simulink library "microgridLibrary"  (R2018b)
settings: Solver=VariableStepAuto  StartTime=0.0  StopTime=10.0  RelTol=1e-3
undefined symbols (not defined in the file): BR, D1, Delta, DiscIntNeverNeededParam, Fn, gcbh, Ion, kv, Lithium, Ls, Rs, sps_rtmsupport, StationData, Ts, Ts_Control, Vn
libraries: powerlib x80, simulink x29, powerlib_meascontrol x28, sps_avr x5, spsDieselMotorModel x3, electricdrivelib x2, re_lib x1
(part 1 of 6)
settings Model: Creator=jlesage  LastModifiedBy=jlesage
settings DebuggingCC: LibraryContextMissingDiagnostic=none
settings SFSimCC: SimUseLocalCustomCode=off
settings RTWCC: RTWUseLocalCustomCode=off

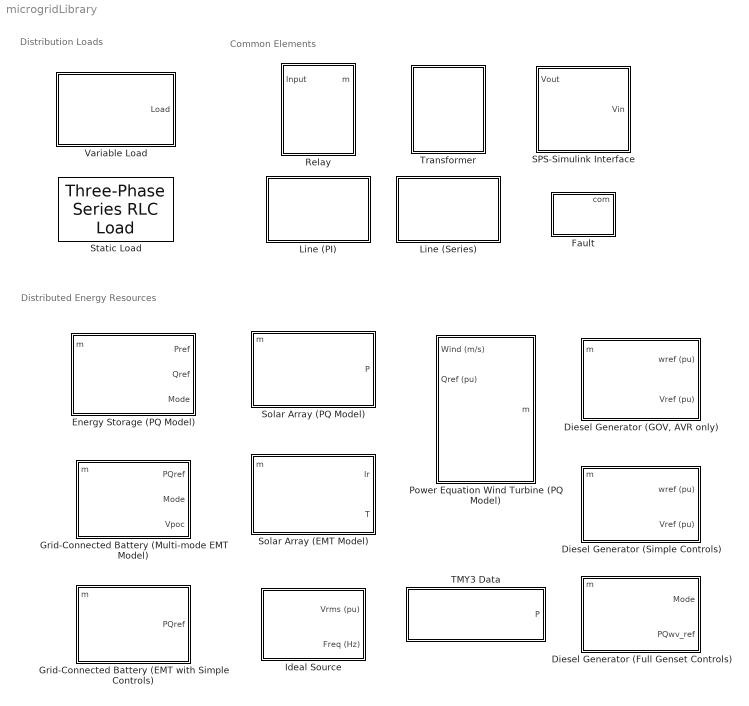
== system microgridLibrary ==
  note: Distribution Loads
  note: Common Elements
  note: Distributed Energy Resources
  Diesel Generator (Full Genset Controls) : Subsystem  VariantControlMode=Label  Variant=on  VariantControl=Variant1  LabelModeActiveChoice=Continuous  mask(Diesel Generator (Full Genset Model)){Pn=1e7, Vn=5000, Fn=60, genType=PQ, PQ0=[0.8 0], Ts=0, copyToDis=on}
      mask prompts: Pn "Generator Rated Power [W]"; Vn "Rated Voltage [V]"; Fn "Rated Frequency [Hz]"; genType "Load Flow Type"; PQ0 "Initial Power, [P0 Q0] [pu]"; Ts "Sample Time [s]"; copyToDis "Copy Load Flow to Discrete"
      mask help:
      | The Diesel Generator block contains a synchronous generator, diesel governor and excitation system to represent the dynamics of a Genset. Additional Genset controls are available for different control tasks, such as PQ control, PV control and VF control.
      |
      | The inputs to the Genset block are Mode (0 - VF control, 1 - PQ control, 2 - PV control)  and the command vector (Pref, Qref, wref, Vref) . The output measurements are contained in a Simulink bus, which can be selected by using the Bus Selector block.
      |
      | Note: The initial generator power must be specified for use for Load Flow analysis.
      mask init:
      | pf = 0.95;
      | 
      | % Extract Initial Active/Reactive Power
      | P0 = PQ0(1);
      | Q0 = PQ0(2);
      | 
      | simulationStatus =  get_param(bdroot,'SimulationStatus');
      | 
      | % The active variant can only be modified at edit-time or very early during
      | % the simulink compile stage. 
      | if any(strcmp(simulationStatus, {'stopped'}))
      |     vssBlk = gcb;
      |     oldVariant = get_param(gcb,'OverrideUsingVariant');
      | 
      |     if Ts == 0
      |         set_param(vssBlk, 'OverrideUsingVariant', 'Continuous');
      |     else
      |         set_param(vssBlk, 'OverrideUsingVariant', 'Discrete');
      |     end
      | end
      | 
      | % Select Load Flow Type
      | genBlock = [gcb '/Continuous/Synchronous Machine'];
      | currentVals = get_param(genBlock,'MaskValues');
      | currentVals{31} = genType;
      | set_param(genBlock,'MaskValues',currentVals);
      | 
      | % Disable Option if Swing Generator Selected
      | currentEnables = get_param(gcb,'MaskEnables');
      | if strcmp(genType,'swing') && Ts == 0
      |     currentEnables{4} = 'on';
      |     currentEnables{5} = 'off';
      | elseif Ts == 0
      |     currentEnables{4} = 'on';
      |     currentEnables{5} = 'on';
      | else
      |     currentEnables{4} = 'off';
      |     currentEnables{5} = 'off';
      | end
      | set_param(gcb,'MaskEnables',currentEnables);
      | 
      | % Copy Load Flow Results to Discrete
      | if copyToDis
      | contGenBlock = [gcb '/Continuous/Synchronous Machine'];
      | contGovBlock = [gcb '/Continuous/Diesel Engine Governor'];
      | contAvrBlock = [gcb '/Continuous/Excitation System'];
      | 
      | disGenBlock = [gcb '/Discrete/Synchronous Machine'];
      | disGovBlock = [gcb '/Discrete/Diesel Engine Governor'];
      | disAvrBlock = [gcb '/Discrete/Excitation System'];
      | 
      | contGenParam = get_param(contGenBlock,'MaskValues');
      | contGovParam = get_param(contGovBlock,'MaskValues');
      | contAvrParam = get_param(contAvrBlock,'MaskValues');
      | 
      | disGenParam = get_param(disGenBlock,'MaskValues');
      | disGovParam = get_param(disGovBlock,'MaskValues');
      | disAvrParam = get_param(disAvrBlock,'MaskValues');
      | 
      | % Overwrite Initial Conditions
      | disGenParam{23} = contGenParam{23};
      | disGovParam{6} = contGovParam{6};
      | disAvrParam{12} = contAvrParam{12};
      | 
      | set_param(disGenBlock,'MaskValues',disGenParam);
      | set_param(disGovBlock,'MaskValues',disGovParam);
      | set_param(disAvrBlock,'MaskValues',disAvrParam);
      | end
      mask TypeOptions genType: swing | PQ
      mask Display:
      | color('black')
      | port_label('input',1,'Mode')
      | port_label('input',2,'PQwvRef')
      | port_label('output',1,'m')
      | port_label('Rconn',1,'A')
      | port_label('Rconn',2,'B')
      | port_label('Rconn',3,'C')
  "Diesel Generator (GOV, AVR only)" : Subsystem  mask(Diesel Generator (Simple)){Pn=1e6, Vn=5000, Fn=60, genType=PQ, PQ0=[0.05 0]}
      mask prompts: Pn "Generator Rated Power [W]"; Vn "Rated Voltage [V]"; Fn "Rated Frequency [Hz]"; genType "Load Flow Type"; PQ0 "Initial Power, [P0 Q0] [pu]"
      mask help:
      | The Diesel Generator block contains a synchronous generator, diesel governor and excitation system to represent the dynamics of a Genset. To inspect the model, look under the block mask (Ctrl + u).
      |
      | The inputs to the basic Diesel generator block are the desired speed reference (in pu) and the desired voltage reference (in pu). The output measurements are contained in a Simulink bus, which can be selected by using the Bus Selector block.
      |
      | Note: The initial generator power must be specified for use for Load Flow analysis.
      mask init:
      | % Extract Initial Active/Reactive Power
      | P0 = PQ0(1);
      | Q0 = PQ0(2);
      | 
      | % Select Load Flow Type
      | genBlock = [gcb '/Synchronous Machine'];
      | currentVals = get_param(genBlock,'MaskValues');
      | currentVals{31} = genType;
      | set_param(genBlock,'MaskValues',currentVals);
      | 
      | % Disable Option if Swing Generator Selected
      | currentEnables = get_param(gcb,'MaskEnables');
      | if strcmp(genType,'swing')
      |     currentEnables{5} = 'off';
      | else
      |     currentEnables{5} = 'on';
      | end
      | set_param(gcb,'MaskEnables',currentEnables);
      mask TypeOptions genType: swing | PQ | PV
      mask Display:
      | %image(imread('diesel.jpg'))
      | color('black')
      | port_label('input',1,'wref (pu)')
      | port_label('input',2,'Vref (pu)')
      | port_label('output',1,'m')
      | port_label('Rconn',1,'A')
      | port_label('Rconn',2,'B')
      | port_label('Rconn',3,'C')
  Diesel Generator (Simple Controls) : Subsystem  VariantControlMode=Label  Variant=on  VariantControl=Variant1  LabelModeActiveChoice=Continuous  mask(Diesel Generator (Simple)){Pn=6e7, Vn=5000, Fn=60, genType=swing, PQ0=[0.4 0], Ts=0, copyToDis=on}
      mask prompts: Pn "Generator Rated Power [W]"; Vn "Rated Voltage [V]"; Fn "Rated Frequency [Hz]"; genType "Load Flow Type"; PQ0 "Initial Power, [P0 Q0] [pu]"; Ts "Sample Time [s]"; copyToDis "Copy Load Flow to Discrete"
      mask help:
      | The Diesel Generator block contains a synchronous generator, diesel governor and excitation system to represent the dynamics of a Genset. To inspect the model, look under the block mask (Ctrl + u).
      |
      | The inputs to the basic Diesel generator block are the desired speed reference (in pu) and the desired voltage reference (in pu). The output measurements are contained in a Simulink bus, which can be selected by using the Bus Selector block.
      |
      | Note: The initial generator power must be specified for use for Load Flow analysis.
      mask init: same as microgridLibrary/Diesel Generator (Full Genset Controls)
      mask TypeOptions genType: swing | PQ
      mask Display:
      | color('black')
      | port_label('input',1,'wref (pu)')
      | port_label('input',2,'Vref (pu)')
      | port_label('output',1,'m')
      | port_label('Rconn',1,'A')
      | port_label('Rconn',2,'B')
      | port_label('Rconn',3,'C')
  Energy Storage (PQ Model) : Subsystem  mask(Grid-connected Energy Storage (PQ Model)){SimMode=Phasor, Vn=5000, Fn=60, PnomkW=500, kWh_Rated=100, Efficiency=96, LimitVec=[90 10], RechargeSOC=11, Precharge=50, autoRecharge=off, Initial_kWh_pc=80, PQvec=[500e3 0]}
      mask prompts: SimMode "Simulation Mode"; Vn "Nominal L-L Voltage [Vrms]"; Fn "Nominal Frequency [Hz]"; PnomkW "Rated Power [kW]"; kWh_Rated "Rated Capacity [kWh]"; Efficiency "Overall System Efficiency [%]"; LimitVec "Upper/Lower Charge Limits [%]"; RechargeSOC "SOC to Recharge [%]"; Precharge "Recharge Rate [% of Rated Power]"; autoRecharge "Enable Auto-Recharge"; Initial_kWh_pc "Initial State-of-Charge [0-100%]"; PQvec "Initial Active/Reactive Cmds"
      mask help:
      | The energy storage block models a generic grid-connected energy storage system (ESS), most commonly a battery system. This is a system-level model that does not contain any power electronics, but is useful for load flow, phasor, and hybrid phasor-EMT simulations. The inputs to this block are the commanded active and reactive power of the ESS. The ESS is assumed to have four quadrent operation. The Mode Input dictates what high-level operation the ESS has: current control (Mode = 1) or voltage control (Mode = 0). Current control is ideal for a grid connected system where you need to specify P,Q commands. Voltage control is necessary if the ESS will be the only system supporting the microgrid in islanded mode.
      |
      | For more detailed ESS models, consider the battery block in the Drives library. Consider using this PQ Model to perform load flow studies and switch to a more detailed model when full EMT studies or more advanced controls are required.
      |
      | Note: The initial active/reactive power commands must be specified for use for Load Flow analysis.
      mask init:
      | % Calculate Initial Conditions
      | Pnom = PnomkW*1e3;
      | P0 = -PQvec(1);  Q0 = -PQvec(2);
      | if abs(P0) > Pnom
      |     P0 = sign(P0)*Pnom;
      | end
      | 
      | % Calculate Q0 given Reactive Power Capability Curve
      | Qlim = sqrt(Pnom^2 - P0^2);
      | if Qlim > abs(Q0)
      |     Q0 = sign(Q0)*Qlim;
      | end
      | 
      | UpChrgLim = LimitVec(1);
      | LowChrgLim = LimitVec(2);
      | if Initial_kWh_pc > UpChrgLim && P0 < 0
      |     P0 = 0; Q0 = 0;
      | elseif Initial_kWh_pc < LowChrgLim && P0 > 0
      |     P0 = 0; Q0 = 0;
      | end
      | 
      | simulationStatus =  get_param(bdroot,'SimulationStatus');
      | 
      | % The active variant can only be modified at edit-time or very early during
      | % the simulink compile stage. 
      | if any(strcmp(simulationStatus, {'stopped'}))
      | 
      | blk = [gcb '/Power Measures'];
      | if strcmp(SimMode,'Phasor')
      |     set_param(blk,'OverrideUsingVariant','Phasor');
      | else
      |     set_param(blk,'OverrideUsingVariant','EMT');
      | end
      | 
      | 
      | end
      mask TypeOptions SimMode: Electromagnetic Transient (EMT) | Phasor
      mask DialogControl Container7 Prompt: Grid Connection Properties
      mask DialogControl Container11 Prompt: Charge/Discharge Controls
      mask DialogControl Container12 Prompt: Initial Conditions
      mask Display: plot(-80,-50,80,50,[0,9,18,24,29,30,29,24,18,9,0,-9,-18,-24,-29,-30,-29,-24,-18,-9,0],[30,29,24,18,9,0,-9,-18,-24,-29,-30,-29,-24,-18,-9,0,9,18,24,29,30],[-50],[0],[50],[0],[45 35 40 40 40],[15 15 15 20 10],[1 2 3 4 5 6 7 8 9 10 11 12 13 14 15 16 17 18 19 20 21].*1.5-15,[0,9,18,24,29,30,29,24,18,9,0,-9,-18,-24,-29,-30,-29,-24,-18,-9,0]./2.4)
  "Fault " : Subsystem  DialogController=POWERSYS.PowerSysDialog  LoadFcn=sps_rtmsupport('LoadFcn',gcbh);  StartFcn=sps_rtmsupport('StartFcn',gcbh);  StopFcn=sps_rtmsupport('StopFcn',gcbh);  mask(Three-Phase Fault){InitialStates=0, FaultA=on, FaultB=on, FaultC=on, GroundFault=on, SwitchTimes=[ 1/60 6/60], External=on, SwitchStatus=NaN, FaultResistance=0.01, GroundResistance=0.001, SnubberResistance=inf, SnubberCapacitance=inf, Measurements=Fault currents}
      mask prompts: InitialStates "Initial status:"; FaultA "Phase A"; FaultB "Phase B"; FaultC "Phase C"; GroundFault "Ground"; SwitchTimes "Switching times (s):"; SwitchStatus "Transition status:"; FaultResistance "Fault resistance Ron (Ohm):"; GroundResistance "Ground resistance Rg (Ohm):"; SnubberResistance "Snubber resistance Rs (Ohm):"; SnubberCapacitance "Snubber capacitance Cs (F):"
      mask help: Implements a fault (short-circuit) between any phase and the ground. When the external switching time mode is selected, a Simulink logical signal is used to control the fault operation.
      mask init:
      | block = gcb;
      | [FaultIcon,FaultA,FaultB,FaultC,GroundResistance,initialA,initialB,initialC,Ts,SwitchTimes,SwitchStatus] = powericon('ThreePhaseFaultInit',block,GroundResistance,SwitchTimes,SwitchStatus,FaultA,FaultB,FaultC,GroundFault,InitialStates,External);
      | powericon('ThreePhaseFaultCback',block);
      settings: CopyFcn=sps_rtmsupport('CopyFcn',gcbh);  DeleteFcn=sps_rtmsupport('DeleteFcn',gcbh);  UndoDeleteFcn=sps_rtmsupport('UndoDeleteFcn',gcbh);  ModelCloseFcn=sps_rtmsupport('ModelCloseFcn',gcbh);  PreSaveFcn=sps_rtmsupport('PreSaveFcn',gcbh);  PostSaveFcn=sps_rtmsupport('PostSaveFcn',gcbh);  NameChangeFcn=sps_rtmsupport('NameChangeFcn',gcbh);  PreCopyFcn=sps_rtmsupport('PreCopyFcn',gcbh);  OpenFcn=sps_rtmsupport('OpenFcn',gcbh, [ 2 3 4 5 7 13]);  CloseFcn=sps_rtmsupport('CloseFcn',gcbh);  PreDeleteFcn=sps_rtmsupport('PreDeleteFcn',gcbh);
      mask Help: helpview(psbhelp)
      mask Callback GroundFault: powericon('ThreePhaseFaultCback',gcb);
      mask Callback External: powericon('ThreePhaseFaultCback',gcb);
      mask TypeOptions Measurements: None | Fault voltages | Fault currents | Fault voltages and currents
      mask DialogControl Container3 Prompt: Fault between:
      mask Display:
      | image(imread(FaultIcon,'bmp'))
      | port_label('LConn', 1, 'A')
      | port_label('LConn', 2, 'B')
      | port_label('LConn', 3, 'C')
  Grid-Connected Battery (EMT with Simple Controls) : Subsystem  mask{Pmod=15, Vnom_dc=480, Bcap=500, Vnom_prim=2400, Fnom=60, Ts=Ts, Ts_Control=Ts_Control}
      mask prompts: Pmod "Scale Battery, Multiplier for 100 kW"; Vnom_dc "Nominal Battery Voltage, V"; Bcap "Battery Capacity, Ah"; Vnom_prim "Nominal Grid Connection L-L Voltage, Vrms"; Fnom "Grid Frequency, Fnom [Hz]"; Ts "Simulation Time Step, Ts [s]"; Ts_Control "Controller Time Step, Ts_Control"
      mask init:
      | Pnom = Pmod*100e3;      % Inverter nominal 3-phase power (VA)
      | Vnom_dc = 480;     % Nominal DC link voltage (V)
      | % Vnom_prim = 25e3;  % Nominal inverter primary line-to-line voltage(Vrms)
      | Vnom_sec= 0.85*Vnom_dc/2/sqrt(2)*sqrt(3); % Nominal inverter secondary line-to-line voltage (Vrms)
      | 
      | TotalLeakage = 0.06;   % Transformer total leakage (pu)
      | Rxf = TotalLeakage/25;
      | Lxf = TotalLeakage;
      | 
      | % Inverter choke RL [Rpu Lpu]
      | Rchoke = 0.15/100;
      | Lchoke = 0.15;
      | Zbase = Vnom_sec^2/Pnom;
      | 
      | % Filter C Parameters
      | Qc = 0.1*Pnom;     % Capacitive reactive power (var)
      | Pc = Qc/50;        % Active power (W)      
      | 
      | Clink = 2 * 3/4 * (Pnom/Fnom*2/Vnom_dc^2); % DC link energy for 3/4 cycle of Pnom
      | 
      | % VDC regulator (VDCreg)
      | Kp_VDCreg = 2;           % Proportional gain
      | Ki_VDCreg = 400;        % Integral gain
      | 
      | Rtot_pu = Rxf + Rchoke; % Feedforward values
      | Ltot_pu = Lxf + Lchoke; % Feedforward values
      | 
      | Kp_Ireg = 0.3;          % Proportional gain
      | Ki_Ireg = 20;           % Integral gain
      mask Display: plot(-80,-50,80,50,[0,9,18,24,29,30,29,24,18,9,0,-9,-18,-24,-29,-30,-29,-24,-18,-9,0],[30,29,24,18,9,0,-9,-18,-24,-29,-30,-29,-24,-18,-9,0,9,18,24,29,30],[-50],[0],[50],[0],[45 35 40 40 40],[15 15 15 20 10],[1 2 3 4 5 6 7 8 9 10 11 12 13 14 15 16 17 18 19 20 21].*1.5-15,[0,9,18,24,29,30,29,24,18,9,0,-9,-18,-24,-29,-30,-29,-24,-18,-9,0]./2.4)
  Grid-Connected Battery (Multi-mode EMT Model) : Subsystem  mask{Pmod=15, Vnom_dc=480, Bcap=500, Vnom_prim=2400, Fnom=60, Ts=Ts, Ts_Control=Ts_Control}
      mask prompts: Pmod "Scale Battery, Multiplier for 100 kW"; Vnom_dc "Nominal Battery Voltage, V"; Bcap "Battery Capacity, Ah"; Vnom_prim "Nominal Grid Connection L-L Voltage, Vrms"; Fnom "Grid Frequency, Fnom [Hz]"; Ts "Simulation Time Step, Ts [s]"; Ts_Control "Controller Time Step, Ts_Control"
      mask init: same as microgridLibrary/Grid-Connected Battery (EMT with Simple Controls)
      mask Display: plot(-80,-50,80,50,[0,9,18,24,29,30,29,24,18,9,0,-9,-18,-24,-29,-30,-29,-24,-18,-9,0],[30,29,24,18,9,0,-9,-18,-24,-29,-30,-29,-24,-18,-9,0,9,18,24,29,30],[-50],[0],[50],[0],[45 35 40 40 40],[15 15 15 20 10],[1 2 3 4 5 6 7 8 9 10 11 12 13 14 15 16 17 18 19 20 21].*1.5-15,[0,9,18,24,29,30,29,24,18,9,0,-9,-18,-24,-29,-30,-29,-24,-18,-9,0]./2.4)
  Ideal Source : Subsystem  DialogController=POWERSYS.PowerSysDialog  LoadFcn=sps_rtmsupport('LoadFcn',gcbh);  StartFcn=sps_rtmsupport('StartFcn',gcbh);  StopFcn=sps_rtmsupport('StopFcn',gcbh);  mask(Three-Phase Source){InternalConnection=Yg, VoltagePhases=off, Voltage=Vn, PhaseAngle=0, Voltage_phases=[25e3 25e3 25e3]/sqrt(3), PhaseAngles_phases=[0 -120 +120], Frequency=Fn, NonIdealSource=off, SpecifyImpedance=off, Resistance=0.8929, Inductance=16.58e-3, ShortCircuitLevel=100e6, BaseVoltage=25e3, XRratio=7, BusType=swing, Pref=10e3, Qref=0, Prefabc=[10e3, 10e3, 10e3], Qrefabc=[0, 0, 0], Qmin=-inf, Qmax=inf}
      mask prompts: InternalConnection "Configuration:"; VoltagePhases "Specify internal voltages for each phase"; Voltage "Phase-to-phase voltage (Vrms):"; PhaseAngle "Phase angle of phase A (degrees):"; Voltage_phases "Line-to-neutral voltages [Va Vb Vc] (Vrms)"; PhaseAngles_phases "Phase angle of line-to-neutral voltages [phia phib phic] (deg)"; Frequency "Frequency (Hz):"; NonIdealSource "Internal"; SpecifyImpedance "Specify short-circuit level parameters"; Resistance "Source resistance (Ohms):"; Inductance "Source inductance (H):"; ShortCircuitLevel "3-phase short-circuit level at base voltage(VA):"; BaseVoltage "Base voltage (Vrms ph-ph):"; XRratio "X/R ratio:"; BusType "Generator type:"; Pref "Active power generation P (W)"; Qref "Reactive power generation Q (var)"; Prefabc "Active power generation [Pa Pb Pc] (W)"; Qrefabc "Reactive power generation [Qa Qb Qc] (var)"; Qmin "Minimum reactive power Qmin or [Qamin,Qbmin Qcmin] (var)"; Qmax "Maximum reactive power Qmax or [Qamax,Qbmax Qcmax] (var)"
      mask help: Three-phase voltage source in series with RL branch.
      mask init:
      | block = gcb;
      | powericon('ThreePhaseSourceCback',block);
      | [s1,s2,s3,s4,g1,g2,g3,g4,g5,g6,s5] = powericon('ThreePhaseSourceIcon',SpecifyImpedance,ShortCircuitLevel,BaseVoltage,Resistance,Inductance,XRratio,InternalConnection,NonIdealSource);
      | powericon('psbloadfunction',block,'goto','Initialize');
      | [Ts, WantBlockChoice,Aa,Pa,Ab,Pb,Ac,Pc] = powericon('ThreePhaseSourceInit',block,Voltage,PhaseAngle,Voltage_phases,PhaseAngles_phases,VoltagePhases);
      | %powericon('SetInternalModels','set',block,WantBlockChoice);
      settings: CopyFcn=sps_rtmsupport('CopyFcn',gcbh); powericon('psbloadfunction',gcb,'goto','UpdateGotoTag');  DeleteFcn=sps_rtmsupport('DeleteFcn',gcbh);  UndoDeleteFcn=sps_rtmsupport('UndoDeleteFcn',gcbh);  ModelCloseFcn=sps_rtmsupport('ModelCloseFcn',gcbh);  PreSaveFcn=sps_rtmsupport('PreSaveFcn',gcbh);  PostSaveFcn=sps_rtmsupport('PostSaveFcn',gcbh);  NameChangeFcn=sps_rtmsupport('NameChangeFcn',gcbh);  PreCopyFcn=sps_rtmsupport('PreCopyFcn',gcbh);  OpenFcn=sps_rtmsupport('OpenFcn',gcbh, [1,2,8,-9,15]);  CloseFcn=sps_rtmsupport('CloseFcn',gcbh);  PreDeleteFcn=sps_rtmsupport('PreDeleteFcn',gcbh);
      mask Help: helpview(psbhelp);
      mask TypeOptions InternalConnection: Y | Yn | Yg
      mask Callback InternalConnection: %powericon('ThreePhaseSourceCback',gcb);
      mask Callback VoltagePhases: powericon('ThreePhaseSourceCback',gcb);
      mask Callback NonIdealSource: powericon('ThreePhaseSourceCback',gcb);
      mask Callback SpecifyImpedance: powericon('ThreePhaseSourceCback',gcb);
      mask TypeOptions BusType: swing | PV | PQ
      mask Callback BusType: powericon('ThreePhaseSourceCback',gcb);
      mask Callback Qmax: sps_rtmsupport('parametereditingmodes',gcbh, [1,2,8,-9,15]);
      mask DialogControl Parameters Prompt: Parameters
      mask DialogControl Container7 Prompt: Source
      mask DialogControl Container6 Prompt: Impedance
      mask DialogControl LoadFlow Prompt: Load Flow
      mask Display:
      | plot(-180,-50,s5,50,s1,s2,s3,s4,[0,9,18,24,29,30,29,24,18,9,0,-9,-18,-24,-29,-30,-29,-24,-18,-9,0]*1.5-45, [30,29,24,18,9,0,-9,-18,-24,-29,-30,-29,-24,-18,-9,0,9,18,24,29,30]*0.8,[-150,-90],[0,0]);
      | plot(g1,g2,g3,g4,g5,g6);
      | plot([1 2 3 4 5 6 7 8 9 10 11 12 13 14 15 16 17 18 19 20 21].*2.5-72, [0,9,18,24,29,30,29,24,18,9,0,-9,-18,-24,-29,-30,-29,-24,-18,-9,0]./3)
  Line (PI) : Subsystem  mask{gauge=500 Kcmil, Freq=60, Length_ft=50, Ratio=3}
      mask prompts: gauge "Line Gauge"; Freq "Nominal Frequency, Hz"; Length_ft "Length, ft"; Ratio "Ratio Impedance, Z0/Z1"
      mask init:
      | Length = 0.0003048*Length_ft; % ft/km
      | 
      | MaskVals = get_param(gcb,'MaskValues');
      | GaugeStr = MaskVals{1};
      | LengthStr = MaskVals{3};
      | 
      | switch gauge
      |     case 1  %500 Kcmil
      |         R0 = 0.0965;        L0 = 3.0372e-04;        
      |     case 2  %350 Kcmil
      |         R0 = 0.1240;        L0 = 3.2461e-04; 
      |     case 3  %4/0 AWG
      |         R0 = 0.2100;        L0 = 3.3156e-04; 
      |     case 4  %3/0 AWG
      |         R0 = 0.2653;        L0 = 3.3800e-04;
      |     case 5  %2/0 AWG
      |         R0 = 0.3346;        L0 = 3.5420e-04; 
      |     case 6  %1/0 AWG
      |         R0 = 0.4199;        L0 = 3.6030e-04;
      | end
      | 
      | % Zero-sequence Parameters
      | R1 = R0/Ratio;
      | L1 = L0/Ratio;
      mask TypeOptions gauge: 500 Kcmil | 350 Kcmil | 4/0 AWG | 3/0 AWG | 2/0 AWG | 1/0 AWG
      mask Display:
      | plot(0,0,1,1,[.20,.20,.80,.80,.90,.80,.80,.20,.20,.10],[.50,.40,.40,.50,.50,.50,.61,.61,.50,.50],[.56,.39],[.55,.55],[.44,.44],[.44,.55],[.53,.50,.50],[.44,.48,.55])
      | 
      | text(0.5,0.75,GaugeStr,'horizontalAlignment', 'center');
      | text(0.5,0.3,[LengthStr ' ft'],'horizontalAlignment', 'center');
      | 
      | 
      | port_label('RConn', 1, 'a')
      | port_label('RConn', 2, 'b')
      | port_label('RConn', 3, 'c')
      | port_label('LConn', 1, 'A')
      | port_label('LConn', 2, 'B')
      | port_label('LConn', 3, 'C')
  Line (Series) : Subsystem  mask{gauge=500 Kcmil, Length=50}
      mask prompts: gauge "Line Gauge"; Length "Length, ft"
      mask init:
      | MaskVals = get_param(gcb,'MaskValues');
      | GaugeStr = MaskVals{1};
      | LengthStr = MaskVals{2};
      | 
      | switch gauge
      |     case 1  %500 Kcmil
      |         R0 = 2.94e-5;       L0 = 9.2575e-8;        
      |     case 2  %350 Kcmil
      |         R0 = 3.78e-5;       L0 = 9.8941e-8; 
      |     case 3  %4/0 AWG
      |         R0 = 6.4e-5;        L0 = 1.03-07; 
      |     case 4  %3/0 AWG
      |         R0 = 7.61e-5;       L0 = 1.05e-7;
      |     case 5  %2/0 AWG
      |         R0 = 1.02e-4;       L0 = 1.0796e-7; 
      |     case 6  %1/0 AWG
      |         R0 = 1.28e-4;       L0 = 1.0982e-7;
      | end
      | 
      | R0 = R0;
      | L0 = L0;
      mask TypeOptions gauge: 500 Kcmil | 350 Kcmil | 4/0 AWG | 3/0 AWG | 2/0 AWG | 1/0 AWG
      mask Display:
      | plot(0,0,1,1,[.20,.20,.80,.80,.90,.80,.80,.20,.20,.10],[.50,.40,.40,.50,.50,.50,.61,.61,.50,.50])
      | 
      | text(0.5,0.75,GaugeStr,'horizontalAlignment', 'center');
      | text(0.5,0.3,[LengthStr ' ft'],'horizontalAlignment', 'center');
      | 
      | 
      | port_label('RConn', 1, 'a')
      | port_label('RConn', 2, 'b')
      | port_label('RConn', 3, 'c')
      | port_label('LConn', 1, 'A')
      | port_label('LConn', 2, 'B')
      | port_label('LConn', 3, 'C')
  Power Equation Wind Turbine (PQ Model) : Subsystem  mask{Unom=15, Umax=25, Umin=5, Pselect=Simple Cubic Power, Vrms=5000, Fnom=60, rp=5, Cp=16/27, rho=1.225, Pnom=500e3, Uvec=[1:1:30], Pvec=[0,0,0,0,21359.3750000000,58193.5000000000,104316.125000000,157104.500000000,213935.875000000,272187.500000000,329236.625000000,382460.500000000,429236.375000000,466941.500000000,492953.125000000,500000,500000,500000,500000,500000,500000,500000,500000,500000,500000,0,0,0,0,0], Tp=0.1, Tq=1, ReactP=30}
      mask prompts: Unom "Nominal Wind Speed [m/s]"; Umax "Maximum Operating Wind [m/s]"; Umin "Minimum Operating Wind [m/s]"; Pselect "Wind Turbine Power Method"; Vrms "Nominal Voltage, Vrms"; Fnom "Nominal Frequency, Hz"; rp "Blade Radius, r [m]"; Cp "Performance Coefficient, Cp"; rho "Air Density, rho [kg/m^3]"; Pnom "Nominal Power, [W]"; Uvec "Wind Vec [m/s]"; Pvec "Power Vec [W]"; Tp "Active Power Dynamics, Tp [s]"; Tq "Reactive Power Dynamics, Tq [s]"; ReactP "Reactive Power Percentage [%]"
      mask help:
      | Simple Wind Turbine that serves as an Active and Reactive Power Source depending on the Wind Power Curve.
      |
      | The Wind Turbine Power Curve can be defined by:
      | - Dimentions of the wind turbine
      | - Simple cubic power curve
      | - Look-up vector from a wind turbine data sheet.
      mask init:
      | A = pi*rp^2;
      | 
      | if Pselect == 1,
      |     Pmax = 1/2*rho*Cp*A*Umax^3;
      | elseif Pselect == 2,
      |     Pmax = Pnom;
      | else
      |     Pmax = max(Pvec);
      | end
      | Qmax = ReactP/100*Pmax;
      mask TypeOptions Pselect: Using Properties | Simple Cubic Power | Look-up Fit
      mask DialogControl Container4 Prompt: General
      mask DialogControl Container9 Prompt: Dimensions
      mask DialogControl Container12 Prompt: Cubic
      mask DialogControl Container7 Prompt: Lookup
      mask DialogControl Container8 Prompt: Dynamics
      mask Display:
      | image(imread('eolienne.bmp'))
      | 
      | color('white')
      | port_label('LConn',1,'A')
      | port_label('LConn',2,'B')
      | port_label('LConn',3,'C')
      | 
      | color('blue')
      | port_label('output',1,'m')
      | port_label('input',1,'Wind (m/s)')
      | port_label('input',2,'Qref')
  Relay : Subsystem
      mask Display:
      | X.p1 = -20;
      | X.p2 = 120;
      | Y.p1 = 0;
      | Y.p2 = 100;
      | X.p3 = [15,15,25,25,15];
      | Y.p3 = [55,45,45,55,55];
      | X.p4 = [75,75,85,85,75];
      | Y.p4 = [55,45,45,55,55];
      | X.p5 = [25,75];
      | Y.p5 = [50,50];
      | X.p6 = [20,20,40,40,60,60,80,80,80,60,60,40,40];
      | Y.p6 = [45,30,30,35,35,30,30,45,30,30,25,25,30];
      | plot(X.p1,Y.p1,X.p2,Y.p2,X.p3,Y.p3,X.p4,Y.p4,X.p5,Y.p5,X.p6,Y.p6)
      | 
      | port_label('input',1','Cmd');
      | port_label('output',1,'m');
      | 
      | port_label('RConn', 1, 'a')
      | port_label('RConn', 2, 'b')
      | port_label('RConn', 3, 'c')
      | port_label('LConn', 1, 'A')
      | port_label('LConn', 2, 'B')
      | port_label('LConn', 3, 'C')
  SPS-Simulink Interface : Subsystem  VariantControlMode=Label  Variant=on  LabelModeActiveChoice=Phasor  mask(SPS-to-Simulink Voltage Interface){replayType=Phasor Replay, Freq=60, kv=kv, Rs=Rs, Ls=Ls, Ts=Ts}
      mask prompts: replayType "Replay Type"; Freq "Nominal Frequency [Hz]"; kv "Voltage Stability Factor, kv"; Rs "Series Resistance, Rs"; Ls "Series Inductance, Ls"; Ts "Sample Time, Ts"
      mask help:
      | This block uses voltage transfer theory to segment a Simscape Power Systems network into subsystems. These subsystems can execute a multiple rates, use Phasor/EMT simulation methods, and run on multiple cores for real-time simulation.
      |
      | Make sure to select the same simulation technique as the powergui setting in the same subsystem.
      mask init:
      | simulationStatus =  get_param(bdroot,'SimulationStatus');
      | 
      | % The active variant can only be modified at edit-time or very early during
      | % the simulink compile stage. 
      | if any(strcmp(simulationStatus, {'stopped'}))
      |     vssBlk = gcb;
      |     freqBlk = [vssBlk '/EMT/Frequency Generator'];
      | 
      |     if strcmp(replayType,'EMT Replay')
      |         set_param(vssBlk, 'OverrideUsingVariant', 'EMT');
      |     else
      |         set_param(vssBlk, 'OverrideUsingVariant', 'Phasor');
      |     end
      |     
      |     if Ts ~= 0
      |         set_param(freqBlk,'OverrideUsingVariant', 'Discrete');
      |     else
      |         set_param(freqBlk, 'OverrideUsingVariant', 'Continuous');
      |     end
      | end
      mask TypeOptions replayType: EMT Replay | Phasor Replay
  Solar Array (EMT Model) : Subsystem  mask{Pmod=2.5, Vnom_prim=25e3, Fnom=60, Ts=Ts, Ts_Control=Ts_Control}
      mask prompts: Pmod "Scale Array, Multiplier for 100 kW"; Vnom_prim "Nominal Grid Connection L-L Voltage, Vrms"; Fnom "Grid Frequency, Fnom [Hz]"; Ts "Simulation Time Step, Ts [s]"; Ts_Control "Controller Time Step, Ts_Control"
      mask init:
      | Pnom = Pmod*100e3;      % Inverter nominal 3-phase power (VA)
      | Vnom_dc = 480;     % Nominal DC link voltage (V)
      | % Vnom_prim = 25e3;  % Nominal inverter primary line-to-line voltage(Vrms)
      | Vnom_sec= 0.85*Vnom_dc/2/sqrt(2)*sqrt(3); % Nominal inverter secondary line-to-line voltage (Vrms)
      | 
      | TotalLeakage = 0.06;   % Transformer total leakage (pu)
      | Rxf = TotalLeakage/25;
      | Lxf = TotalLeakage;
      | 
      | % Inverter choke RL [Rpu Lpu]
      | Rchoke = 0.15/100;
      | Lchoke = 0.15;
      | Zbase = Vnom_sec^2/Pnom;
      | 
      | % Filter C Parameters
      | Qc = 0.1*Pnom;     % Capacitive reactive power (var)
      | Pc = Qc/50;        % Active power (W)      
      | 
      | Clink = 2 * 3/4 * (Pnom/Fnom*2/Vnom_dc^2); % DC link energy for 3/4 cycle of Pnom
      | 
      | % MPPT Control (Perturb & Observe Algorithm)
      | Increment_MPPT = 0.01;     % Increment value used to increase/decrease Vdc_ref
      | Limits_MPPT = [ 1.25*Vnom_dc 0.75*Vnom_dc ]; % Upper & Lower limit for Vdc_ref (V)
      | 
      | % VDC regulator (VDCreg)
      | Kp_VDCreg = 2;           % Proportional gain
      | Ki_VDCreg = 400;        % Integral gain
      | 
      | Rtot_pu = Rxf + Rchoke; % Feedforward values
      | Ltot_pu = Lxf + Lchoke; % Feedforward values
      | 
      | Kp_Ireg = 0.3;          % Proportional gain
      | Ki_Ireg = 20;           % Integral gain
      mask Display:
      | image(imread('panel.jpg'))
      | color('yellow')
      | port_label('input',1,'Ir')
      | port_label('input',2,'T')
      | port_label('output',1,'m')
      | port_label('output',1,'m')
      | port_label('Rconn',1,'A')
      | port_label('Rconn',2,'B')
      | port_label('Rconn',3,'C')
  Solar Array (PQ Model) : Subsystem  mask(Grid-Connected PV Array (PQ Model)){Vn=5000, Fn=60, P0=500e3}
      mask prompts: Vn "Nominal L-L Voltage [Vrms]"; Fn "Nominal Frequency [Hz]"; P0 "Initial Power [W]"
      mask help:
      | This block models a grid-connected solar array using the Three-Phase Dynamic Load block. This is a system-level model that does not contain any power electronics, but is useful for load flow, phasor, and hybrid phasor-EMT simulations. The input to this block is the power output of the grid connected PV array, not irradiance.
      |
      | For more detailed PV models, consider the PV Array block in the Renewables library. Consider using this PQ Model to perform load flow studies and switch to a more detailed model when full EMT studies are required.
      |
      | Note: The array power must be specified for use for Load Flow analysis.
      mask init:
      | % P0 = Irr0*TotalArea*Efficiency/100;
      | P0 = -P0;
      mask Display:
      | image(imread('PV_Farm.jpg'))
      | color('white')
      | port_label('input',1,'P')
      | port_label('output',1,'m')
      | port_label('Rconn',1,'A')
      | port_label('Rconn',2,'B')
      | port_label('Rconn',3,'C')
  Static Load : powerlib/Elements/Three-Phase Series RLC Load  LConnTagsString=A|B|C  Configuration=Y (grounded)  NominalVoltage=5000  Vabc=[1e3 1e3 1e3]  Vabcp=[1e3 1e3 1e3]  NominalFrequency=60  UnbalancedPower=off  ActivePower=500e3  InductivePower=0  CapacitivePower=0  Pabc=[10e3 9e3 11e3]  QLabc=[100 90 110]  QCabc=[100 90 110]  Pabcp=[10e3 9e3 11e3]  QLabcp=[100 90 110]  QCabcp=[100 90 110]  Measurements=None  LoadType=constant Z
      settings: SourceProductName=Simscape Electrical
  TMY3 Data : Subsystem  mask(TMY3 -to- Power){SortByState=on, ListNum_State=Dallas-Fort Worth Intl AP, TX, ListNum_Name=Rock Springs Arpt [Green River - UO], WY, IrradianceType=Global Horizontal Irradiance (Wh/m2), TotalArea=3000, Efficiency=20, PlotData_On=off}
      mask prompts: SortByState "Sort site name by state:"; TotalArea "Solar panels total area (m2):"; Efficiency "Overall system efficiency (%):"; PlotData_On "Plot meteorological data"
      mask help:
      | Convert TMY3 solar irradiance data to Power.
      |
      | TMY3 are data files for the typical meteorological year (TMY) data sets
      | derived from the 1961-1990 and 1991-2005 National Solar Radiation
      | Data Base (NSRDB) archives. The files contain hourly values of solar radiation and meteorological elements for a 1-year period.
      |
      | TMY3 files have been produced by NREL's Electric Systems Center under
      | the Solar Resource Characterization Project, which is funded and
      | monitored by the U.S. Department of Energy's Energy Efficiency and
      | Renewable Energy Office.
      |
      | Look Under Mask for additionnal information
      mask init:
      | BlockName=gcb;
      | % Mask parameters visibility:
      | %
      | MV = get_param(BlockName,'MaskVisibilities');
      | MV{3}='off';
      | if SortByState==1
      | 	MV{2}='on';
      |     MV{3}='off';
      |     str_NameState=ListNum_State;
      | else
      |     MV{2}='off';
      |     MV{3}='on';
      |     str_NameState=ListNum_Name;
      | end
      | set_param(BlockName,'MaskVisibilities',MV)
      | %
      | load StationData_NEW
      | max=size(StationData,2);
      | for i=1:max
      |     if strcmp([StationData(i).Name{1}, ', ', StationData(i).State{1}],str_NameState)
      |        Index=StationData(i).NumberByState;
      |     end
      | end
      | if IrradianceType==1
      |     IrradianceTable=StationData(Index).GHIWm2;
      | else
      |     IrradianceTable=StationData(Index).DNIWm2;
      | end
      | if PlotData_On==1
      |     h2=figure;
      |     set(h2,'Name',[StationData(Index).Name{1}, ', ', StationData(Index).State{1}]);
      |     ScreenS=get(0,'Screensize');
      |     set(h2,'Position',[ScreenS(3)/14 ScreenS(4)/12 ScreenS(3)/2.4 ScreenS(4)/1.25])
      |     subplot(3,1,1)
      |     plot([1:size(StationData(Index).GHIWm2,1)]',StationData(Index).GHIWm2)
      |     title('Global Horizontal Irradiance')
      |     ylabel('Wh/m2')
      |     grid
      |     subplot(3,1,2)
      |     plot([1:size(StationData(Index).DHIWm2,1)]',StationData(Index).DHIWm2)
      |     title('Diffuse Horizontal Irradiance')
      |     ylabel('Wh/m2')
      |     grid
      |     subplot(3,1,3)
      |     plot([1:size(StationData(Index).DNIWm2,1)]',StationData(Index).DNIWm2)
      |     title('Direct Normal Irradiance')
      |     ylabel('Wh/m2')
      |     xlabel('Time of the Year in Hours')
      |     %
      |     h3=figure;
      |     set(h3,'Name',[StationData(Index).Name{1}, ', ', StationData(Index).State{1}]);
      |     ScreenS=get(0,'Screensize');
      |     set(h3,'Position',[ScreenS(3)/2 ScreenS(4)/12 ScreenS(3)/2.4 ScreenS(4)/1.25])
      |     subplot(2,1,1)
      |     plot([1:size(StationData(Index).Temperature,1)]',StationData(Index).Temperature)
      |     title('Temperature')
      |     ylabel('C')
      |     grid
      |     subplot(2,1,2)
      |     plot([1:size(StationData(Index).WindSpeed,1)]',StationData(Index).WindSpeed)
      |     title('Wind Speed')
      |     ylabel('m/s')
      |     grid
      |     xlabel('Time of the Year in Hours')
      |     set_param(BlockName,'PlotData_On', 'off')
      | end
      mask TypeOptions ListNum_State: Birmingham Municipal AP, AL | Huntsville Intl/Jones Field, AL | Mobile Regional AP, AL | Montgomery Dannelly Field, AL | Fort Smith Regional AP, AR | Little Rock Adams Field, AR | Phoenix Sky Harbor Intl AP, AZ | Prescott Love Field, AZ | Tucson International AP, AZ | Arcata Airport, CA | Bakersfield Meadows Field, CA | Bishop Airport, CA | Daggett Barstow-Daggett AP, CA | Fresno Yosemite Intl AP, CA | Long Beach Daugherty Fld, CA | Los Angeles Intl Arpt, CA | Redding Municipal Arpt, CA | Sacramento Executive Arpt, CA | San Diego Lindbergh Field, CA | San Francisco Intl AP, CA | Santa Barbara Municipal AP, CA | Santa Maria Public Arpt, CA | Stockton Metropolitan Arpt, CA | Alamosa San Luis Valley Rgnl, CO | Colorado Springs Muni AP, CO | Denver Intl AP, CO | Grand Junction Walker Field, CO | Limon, CO | Pueblo Memorial AP, CO | Bridgeport Sikorsky Memorial, CT | Hartford Bradley Intl AP, CT | Wilmington New Castle Cnty AP, DE | Daytona Beach Intl AP, FL | Fort Myers Page Field, FL | Gainesville Regional AP, FL | Jacksonville Intl Arpt, FL | Key West Intl Arpt, FL | Miami Intl AP, FL | Orlando Intl Arpt, FL | Pensacola Regional AP, FL | Tallahassee Regional AP [ISIS], FL | Tampa International AP, FL | Vero Beach Municipal Arpt, FL | West Palm Beach Intl Arpt, FL | Athens Ben Epps AP, GA | Atlanta Hartsfield Intl AP, GA | Augusta Bush Field, GA | Columbus Metropolitan Arpt, GA | Macon Middle Ga Regional AP, GA | Savannah Intl AP, GA | Hilo International AP, HI | Honolulu Intl Arpt, HI | Kahului Airport, HI | Lihue Airport, HI | Boise Air Terminal [UO], ID | Lewiston Nez Perce Cnty AP, ID | Pocatello Regional AP, ID | Chicago Ohare Intl AP, IL | Moline Quad City Intl AP, IL | Peoria Greater Peoria AP, IL | Rockford Greater Rockford AP, IL | Springfield Capital AP, IL | Evansville Regional AP, IN | Fort Wayne Intl AP, IN | Indianapolis Intl AP, IN | South Bend Michiana Rgnl AP, IN | Des Moines Intl AP, IA | Dubuque Regional AP, IA | Mason City Municipal Arpt, IA | Sioux City Sioux Gateway AP, IA | Waterloo Municipal AP, IA | Concordia Blosser Muni AP, KS | Dodge City Regional AP, KS | Goodland Renner Field, KS | Russell Municipal AP, KS | Topeka Municipal AP, KS | Wichita Mid-Continent AP, KS | Cincinnati Northern Ky AP, KY | Jackson Julian Carroll AP, KY | Lexington Bluegrass AP, KY | Louisville Standiford Field, KY | Paducah Barkley Regional AP, KY | Baton Rouge Ryan Arpt, LA | Lake Charles Regional Arpt, LA | New Orleans Intl Arpt, LA | Shreveport Regional Arpt, LA | Bangor International AP, ME | Caribou Municipal Arpt, ME | Portland Intl Jetport, ME | Baltimore Blt-Washngtn Int'l, MD | Boston Logan Int'l Arpt, MA | Worchester Regional Arpt, MA | Alpena County Regional AP, MI | Detroit City Airport, MI | Detroit Metropolitan Arpt, MI | Flint Bishop Intl Arpt, MI | Grand Rapids Kent County Int', MI | Houghton Lake Roscommon Co Ar, MI | Lansing Capital City Arpt, MI | Muskegon County Arpt, MI | Sault Ste Marie Sanderson Fie, MI | Traverse City Cherry Capital, MI | Duluth International Arpt, MN | International Falls Intl AP, MN | Minneapolis-St Paul Int'l Arp, MN | Rochester International Arpt, MN | St Cloud Regional Arpt, MN | Jackson International AP, MS | Meridian Key Field, MS | Tupelo C D Lemons Arpt, MS | Columbia Regional Airport, MO | Kansas City Int'l Arpt, MO | Springfield Regional Arpt, MO | St Louis Lambert Int'l Arpt, MO | St Louis Spirit of St Louis Airport, MO | Billings Logan Int'l Arpt, MT | Glasgow Intl Arpt, MT | Great Falls Intl Arpt, MT | Havre City-County AP, MT | Helena Regional Airport, MT | Kalispell Glacier Pk Int'l Ar, MT | Missoula International AP, MT | Grand Island Central NE Regio, NE | Lincoln Municipal Arpt, NE | Norfolk Karl Stefan Mem Arpt, NE | North Platte Regional AP, NE | Omaha Eppley Airfield, NE | Scottsbluff W B Heilig Field, NE | Valentine Miller Field, NE | Ely Yelland Field, NV | Las Vegas McCarran Intl AP, NV | Lovelock Derby Field, NV | Mercury Desert Rock AP [SURFRAD], NV | Reno Tahoe International AP, NV | Tonopah Airport, NV | Winnemucca Municipal Arpt, NV | Concord Municipal Arpt, NH | Atlantic City Intl AP, NJ | Newark International Arpt, NJ | Albuquerque Intl Arpt [ISIS], NM | Gallup Sen Clarke Fld, NM | Roswell Industrial Air Park, NM | Albany County AP, NY | Binghamton Edwin A Link Field, NY | Buffalo Niagara Intl AP, NY | Islip Long Isl MacArthur AP, NY | Massena AP, NY | New York J F Kennedy Int'l Ar, NY | New York Laguardia Arpt, NY | Rochester Greater Rochester I, NY | Syracuse Hancock Int'l Arpt, NY | Asheville Regional Arpt, NC | Charlotte Douglas Intl Arpt, NC | Greensboro Piedmont Triad Int, NC | Raleigh Durham International, NC | Wilmington International Arpt, NC | Bismarck Municipal Arpt [ISIS], ND | Fargo Hector International AP, ND | Minot FAA AP, ND | Williston Sloulin Intl AP, ND | Akron Akron-Canton Reg AP, OH | Cleveland Hopkins Intl AP, OH | Columbus Port Columbus Intl A, OH | Dayton International Airport, OH | Mansfield Lahm Municipal Arpt, OH | Toledo Express Airport, OH | Youngstown Regional Airport, OH | Oklahoma City Will Rogers Wor, OK | Tulsa International Airport, OK | Astoria Regional Airport, OR | Burns Municipal Arpt [UO], OR | Eugene Mahlon Sweet Arpt [UO], OR | Medford Rogue Valley Intl AP [Ashland - UO], OR | Pendleton E Or Regional AP, OR | Salem McNary Field, OR | Allentown Lehigh Valley Intl, PA | Bradford Regional AP, PA | Erie International AP, PA | Middletown Harrisburg Intl AP, PA | Philadelphia International AP, PA | Pittsburgh International AP, PA | Wilkes-Barre Scranton Intl AP, PA | Williamsport Regional AP, PA | Providence T F Green State Ar, RI | Charleston Intl Arpt, SC | Columbia Metro Arpt, SC | Greer Greenv'l-Spartanbrg AP, SC | Aberdeen Regional Arpt, SD | Huron Regional Arpt, SD | Pierre Municipal AP, SD | Rapid City Regional Arpt, SD | Sioux Falls Foss Field, SD | Bristol Tri City Airport, TN | Chattanooga Lovell Field AP, TN | Knoxville McGhee Tyson AP, TN | Memphis International AP, TN | Nashville International AP, TN | Abilene Regional AP [UT], TX | Amarillo International AP [Canyon - UT], TX | Austin Mueller Municipal AP [UT], TX | Brownsville S Padre Isl Intl, TX | Corpus Christi Intl Arpt [UT], TX | Dallas-Fort Worth Intl AP, TX | El Paso International AP [UT], TX | Houston Bush Intercontinental, TX | Lubbock International AP, TX | Lufkin Angelina Co, TX | Midland International AP, TX | Port Arthur Jefferson County, TX | San Angelo Mathis Field, TX | San Antonio Intl AP, TX | Victoria Regional AP, TX | Waco Regional AP, TX | Cedar City Municipal AP, UT | Salt Lake City Int'l Arpt [ISIS], UT | Burlington International AP, VT | Lynchburg Regional Arpt, VA | Norfolk International AP, VA | Richmond International AP, VA | Roanoke Regional AP, VA | Washington DC Dulles Int'l Ar [Sterling - ISIS], VA | Washington DC Reagan AP, VA | Olympia Airport, WA | Quillayute State Airport, WA | Seattle Seattle-Tacoma Intl A, WA | Spokane International AP [Cheney - UO], WA | Stampede Pass, WA | Yakima Air Terminal, WA | Beckley Raleigh Co Mem AP, WV | Charleston Yeager Arpt, WV | Elkins Elkins-Randolph Co Arp, WV | Huntington Tri-State Arpt, WV | Eau Claire County AP, WI | Green Bay Austin Straubel Int, WI | La Crosse Municipal Arpt, WI | Madison Dane Co Regional Arpt [ISIS], WI | Milwaukee Mitchell Intl AP, WI | Casper Natrona Co Intl AP, WY | Cheyenne Municipal Arpt, WY | Lander Hunt Field, WY | Rock Springs Arpt [Green River - UO], WY | Sheridan County Arpt, WY
      mask TypeOptions ListNum_Name: Aberdeen Regional Arpt, SD | Abilene Regional AP [UT], TX | Akron Akron-Canton Reg AP, OH | Alamosa San Luis Valley Rgnl, CO | Albany County AP, NY | Albuquerque Intl Arpt [ISIS], NM | Allentown Lehigh Valley Intl, PA | Alpena County Regional AP, MI | Amarillo International AP [Canyon - UT], TX | Arcata Airport, CA | Asheville Regional Arpt, NC | Astoria Regional Airport, OR | Athens Ben Epps AP, GA | Atlanta Hartsfield Intl AP, GA | Atlantic City Intl AP, NJ | Augusta Bush Field, GA | Austin Mueller Municipal AP [UT], TX | Bakersfield Meadows Field, CA | Baltimore Blt-Washngtn Int'l, MD | Bangor International AP, ME | Baton Rouge Ryan Arpt, LA | Beckley Raleigh Co Mem AP, WV | Billings Logan Int'l Arpt, MT | Binghamton Edwin A Link Field, NY | Birmingham Municipal AP, AL | Bishop Airport, CA | Bismarck Municipal Arpt [ISIS], ND | Boise Air Terminal [UO], ID | Boston Logan Int'l Arpt, MA | Bradford Regional AP, PA | Bridgeport Sikorsky Memorial, CT | Bristol Tri City Airport, TN | Brownsville S Padre Isl Intl, TX | Buffalo Niagara Intl AP, NY | Burlington International AP, VT | Burns Municipal Arpt [UO], OR | Caribou Municipal Arpt, ME | Casper Natrona Co Intl AP, WY | Cedar City Municipal AP, UT | Charleston Intl Arpt, SC | Charleston Yeager Arpt, WV | Charlotte Douglas Intl Arpt, NC | Chattanooga Lovell Field AP, TN | Cheyenne Municipal Arpt, WY | Chicago Ohare Intl AP, IL | Cincinnati Northern Ky AP, KY | Cleveland Hopkins Intl AP, OH | Colorado Springs Muni AP, CO | Columbia Metro Arpt, SC | Columbia Regional Airport, MO | Columbus Metropolitan Arpt, GA | Columbus Port Columbus Intl A, OH | Concord Municipal Arpt, NH | Concordia Blosser Muni AP, KS | Corpus Christi Intl Arpt [UT], TX | Daggett Barstow-Daggett AP, CA | Dallas-Fort Worth Intl AP, TX | Dayton International Airport, OH | Daytona Beach Intl AP, FL | Denver Intl AP, CO | Des Moines Intl AP, IA | Detroit City Airport, MI | Detroit Metropolitan Arpt, MI | Dodge City Regional AP, KS | Dubuque Regional AP, IA | Duluth International Arpt, MN | Eau Claire County AP, WI | El Paso International AP [UT], TX | Elkins Elkins-Randolph Co Arp, WV | Ely Yelland Field, NV | Erie International AP, PA | Eugene Mahlon Sweet Arpt [UO], OR | Evansville Regional AP, IN | Fargo Hector International AP, ND | Flint Bishop Intl Arpt, MI | Fort Myers Page Field, FL | Fort Smith Regional AP, AR | Fort Wayne Intl AP, IN | Fresno Yosemite Intl AP, CA | Gainesville Regional AP, FL | Gallup Sen Clarke Fld, NM | Glasgow Intl Arpt, MT | Goodland Renner Field, KS | Grand Island Central NE Regio, NE | Grand Junction Walker Field, CO | Grand Rapids Kent County Int', MI | Great Falls Intl Arpt, MT | Green Bay Austin Straubel Int, WI | Greensboro Piedmont Triad Int, NC | Greer Greenv'l-Spartanbrg AP, SC | Hartford Bradley Intl AP, CT | Havre City-County AP, MT | Helena Regional Airport, MT | Hilo International AP, HI | Honolulu Intl Arpt, HI | Houghton Lake Roscommon Co Ar, MI | Houston Bush Intercontinental, TX | Huntington Tri-State Arpt, WV | Huntsville Intl/Jones Field, AL | Huron Regional Arpt, SD | Indianapolis Intl AP, IN | International Falls Intl AP, MN | Islip Long Isl MacArthur AP, NY | Jackson International AP, MS | Jackson Julian Carroll AP, KY | Jacksonville Intl Arpt, FL | Kahului Airport, HI | Kalispell Glacier Pk Int'l Ar, MT | Kansas City Int'l Arpt, MO | Key West Intl Arpt, FL | Knoxville McGhee Tyson AP, TN | La Crosse Municipal Arpt, WI | Lake Charles Regional Arpt, LA | Lander Hunt Field, WY | Lansing Capital City Arpt, MI | Las Vegas McCarran Intl AP, NV | Lewiston Nez Perce Cnty AP, ID | Lexington Bluegrass AP, KY | Lihue Airport, HI | Limon, CO | Lincoln Municipal Arpt, NE | Little Rock Adams Field, AR | Long Beach Daugherty Fld, CA | Los Angeles Intl Arpt, CA | Louisville Standiford Field, KY | Lovelock Derby Field, NV | Lubbock International AP, TX | Lufkin Angelina Co, TX | Lynchburg Regional Arpt, VA | Macon Middle Ga Regional AP, GA | Madison Dane Co Regional Arpt [ISIS], WI | Mansfield Lahm Municipal Arpt, OH | Mason City Municipal Arpt, IA | Massena AP, NY | Medford Rogue Valley Intl AP [Ashland - UO], OR | Memphis International AP, TN | Mercury Desert Rock AP [SURFRAD], NV | Meridian Key Field, MS | Miami Intl AP, FL | Middletown Harrisburg Intl AP, PA | Midland International AP, TX | Milwaukee Mitchell Intl AP, WI | Minneapolis-St Paul Int'l Arp, MN | Minot FAA AP, ND | Missoula International AP, MT | Mobile Regional AP, AL | Moline Quad City Intl AP, IL | Montgomery Dannelly Field, AL | Muskegon County Arpt, MI | Nashville International AP, TN | New Orleans Intl Arpt, LA | New York J F Kennedy Int'l Ar, NY | New York Laguardia Arpt, NY | Newark International Arpt, NJ | Norfolk International AP, VA | Norfolk Karl Stefan Mem Arpt, NE | North Platte Regional AP, NE | Oklahoma City Will Rogers Wor, OK | Olympia Airport, WA | Omaha Eppley Airfield, NE | Orlando Intl Arpt, FL | Paducah Barkley Regional AP, KY | Pendleton E Or Regional AP, OR | Pensacola Regional AP, FL | Peoria Greater Peoria AP, IL | Philadelphia International AP, PA | Phoenix Sky Harbor Intl AP, AZ | Pierre Municipal AP, SD | Pittsburgh International AP, PA | Pocatello Regional AP, ID | Port Arthur Jefferson County, TX | Portland Intl Jetport, ME | Prescott Love Field, AZ | Providence T F Green State Ar, RI | Pueblo Memorial AP, CO | Quillayute State Airport, WA | Raleigh Durham International, NC | Rapid City Regional Arpt, SD | Redding Municipal Arpt, CA | Reno Tahoe International AP, NV | Richmond International AP, VA | Roanoke Regional AP, VA | Rochester Greater Rochester I, NY | Rochester International Arpt, MN | Rock Springs Arpt [Green River - UO], WY | Rockford Greater Rockford AP, IL | Roswell Industrial Air Park, NM | Russell Municipal AP, KS | Sacramento Executive Arpt, CA | Salem McNary Field, OR | Salt Lake City Int'l Arpt [ISIS], UT | San Angelo Mathis Field, TX | San Antonio Intl AP, TX | San Diego Lindbergh Field, CA | San Francisco Intl AP, CA | Santa Barbara Municipal AP, CA | Santa Maria Public Arpt, CA | Sault Ste Marie Sanderson Fie, MI | Savannah Intl AP, GA | Scottsbluff W B Heilig Field, NE | Seattle Seattle-Tacoma Intl A, WA | Sheridan County Arpt, WY | Shreveport Regional Arpt, LA | Sioux City Sioux Gateway AP, IA | Sioux Falls Foss Field, SD | South Bend Michiana Rgnl AP, IN | Spokane International AP [Cheney - UO], WA | Springfield Capital AP, IL | Springfield Regional Arpt, MO | St Cloud Regional Arpt, MN | St Louis Lambert Int'l Arpt, MO | St Louis Spirit of St Louis Airport, MO | Stampede Pass, WA | Stockton Metropolitan Arpt, CA | Syracuse Hancock Int'l Arpt, NY | Tallahassee Regional AP [ISIS], FL | Tampa International AP, FL | Toledo Express Airport, OH | Tonopah Airport, NV | Topeka Municipal AP, KS | Traverse City Cherry Capital, MI | Tucson International AP, AZ | Tulsa International Airport, OK | Tupelo C D Lemons Arpt, MS | Valentine Miller Field, NE | Vero Beach Municipal Arpt, FL | Victoria Regional AP, TX | Waco Regional AP, TX | Washington DC Dulles Int'l Ar [Sterling - ISIS], VA | Washington DC Reagan AP, VA | Waterloo Municipal AP, IA | West Palm Beach Intl Arpt, FL | Wichita Mid-Continent AP, KS | Wilkes-Barre Scranton Intl AP, PA | Williamsport Regional AP, PA | Williston Sloulin Intl AP, ND | Wilmington International Arpt, NC | Wilmington New Castle Cnty AP, DE | Winnemucca Municipal Arpt, NV | Worchester Regional Arpt, MA | Yakima Air Terminal, WA | Youngstown Regional Airport, OH
      mask TypeOptions IrradianceType: Global Horizontal Irradiance (Wh/m2) | Direct Normal Irradiance (Wh/m2)
      mask DialogControl Control2 Prompt: Site name:
      mask DialogControl Control3 Prompt: Choose irradiance type:
      mask Display: disp([StationData(Index).Name{1},', ',StationData(Index).State{1}])
  Transformer : Subsystem  mask{kS=225, Freq=60, Vp=4160, Vs=460, Zperc=5.18, Ratio=2.5}
      mask prompts: kS "Nominal Power, kVA"; Freq "Nominal Frequency, Hz"; Vp "Primary L-L Voltage, Vrms"; Vs "Secondary L-L Voltage, Vrms"; Zperc "Impedance - Z, %"; Ratio "X/R Ratio"
      mask init:
      | S = kS*1000;
      | Z = Zperc/100;
      mask Display:
      | plot(-180,-220,180,220,[-100,-40],[0,0],[100,40],[0,0],[2 42 74 94 100 90 66 30 0 2 42 74 94 100 90 66 30 0 2 42 74 94 100 90 66 30 0 2 42 74 94 100 90 66 30 0]*.4-55,[-45 -45 -34 -17 3 22 38 48 50 50 55 66 83 103 122 138 148 150 150 155 166 183 203 222 238 248 250 250 255 266 283 303 322 338 348 348]*0.5-75,[2 42 74 94 100 90 66 30 0 2 42 74 94 100 90 66 30 0 2 42 74 94 100 90 66 30 0 2 42 74 94 100 90 66 30 0]*-.4+55,[-45 -45 -34 -17 3 22 38 48 50 50 55 66 83 103 122 138 148 150 150 155 166 183 203 222 238 248 250 250 255 266 283 303 322 338 348 348]*0.5-75)
      | 
      | 
      | port_label('RConn', 1, 'a')
      | port_label('RConn', 2, 'b')
      | port_label('RConn', 3, 'c')
      | port_label('LConn', 1, 'A')
      | port_label('LConn', 2, 'B')
      | port_label('LConn', 3, 'C')
  Variable Load : Subsystem  mask(Variable Load (PQ Model)){Vn=5000, Fn=60, PF=1, Load0=200e3}
      mask prompts: Vn "Nominal L-L Voltage [Vrms]"; Fn "Nominal Frequency [Hz]"; PF "Power Factor [0 to 1]"; Load0 "Initial Load [W]"
      mask help:
      | The Variable Load block is a lumped approximation for a distribution feeder. For non-unity power factor loads, the input (active power) is scaled accordingly to generate a desired load.
      |
      | Note: The initial input load must be specified for use for Load Flow analysis.
      mask init:
      | P0 = Load0;
      | Q0 = Load0*sqrt(1/PF-1);
      mask Display:
      | image(imread('Residential.jpg'))
      | color('white')
      | port_label('input',1,'Load')
      | port_label('Rconn',1,'A')
      | port_label('Rconn',2,'B')
      | port_label('Rconn',3,'C')
